simulink model "deltaM"  (Simulink 5.0)
settings: Solver=ode45  StartTime=0.0  StopTime=3  RelTol=1e-3
libraries: dspbuff3 x2, dspwin32 x2, dsparch4 x1
settings Model: LastModifiedBy=Daiming Qu

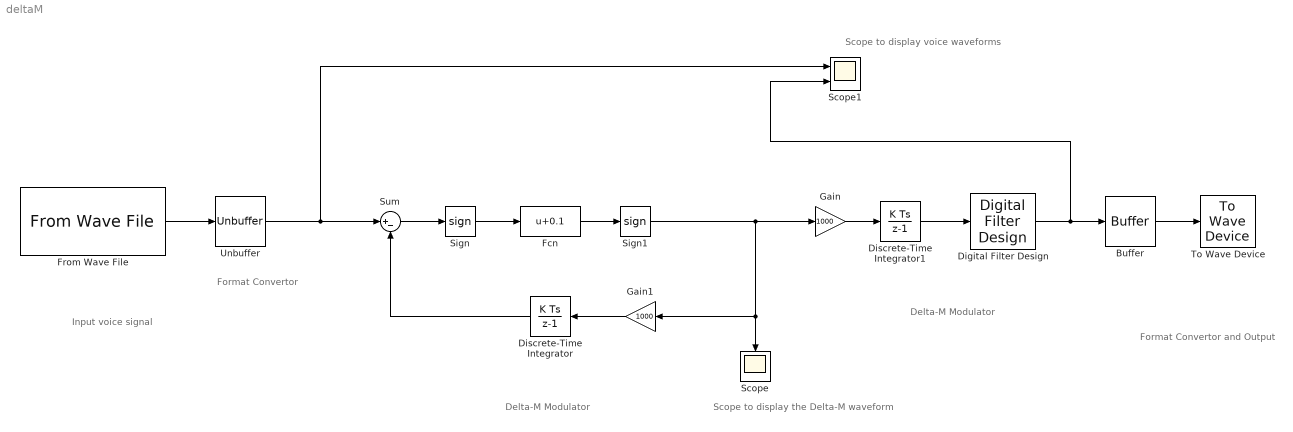
== system deltaM ==
  note: Format Convertor
  note: Scope to display voice waveforms
  note: Scope to display the
      | Delta-M waveform
  note: Format Convertor and Output
  note: Input voice signal
  note: Delta-M Modulator
  note: Delta-M Modulator
  Buffer : dspbuff3/Buffer  N=256  V=0  ic=0
  Digital Filter Design : dsparch4/Digital Filter Design
  Discrete-Time Integrator : DiscreteIntegrator  Orientation=left  SampleTime=-1
  Discrete-Time Integrator1 : DiscreteIntegrator  SampleTime=-1
  Fcn : Fcn  Expr=u+0.1
  From Wave File : dspwin32/From Wave File  FileName=speech_dian.wav  SamplesPerFrame=256  MinBufSize=256  dType=Double
  Gain : Gain  Gain=1000  SaturateOnIntegerOverflow=on
      settings: AttributesFormatString=Gain= %<Gain>
  Gain1 : Gain  Orientation=left  Gain=1000  SaturateOnIntegerOverflow=on
      settings: AttributesFormatString=Gain= %<Gain>
  Scope : Scope
      settings: Orientation=down  TimeRange=0.0004096000000011202  YMin=310.197  YMax=311.835
  Scope1 : Scope  NumInputPorts=2
      settings: TimeRange=10  YMin=-0.75~-0.75  YMax=1~0.75  SampleInput=on
  Sign : Signum
  Sign1 : Signum
  Sum : Sum  Inputs=|+-  SaturateOnIntegerOverflow=on
  To Wave Device : dspwin32/To Wave Device  bufDuration=2  initDelay=0.1  useDefaultDevice=on  userDeviceID=SoundMAX Digital Audio  enable24Bit=off
  Unbuffer : dspbuff3/Unbuffer  ic=0
  wires:
  Sum/1 -> Sign/1
  Discrete-Time Integrator/1 -> Sum/2
  Buffer/1 -> To Wave Device/1
  Discrete-Time Integrator1/1 -> Digital Filter Design/1
  Digital Filter Design/1 -> Buffer/1, Scope1/2
  Unbuffer/1 -> Sum/1, Scope1/1
  From Wave File/1 -> Unbuffer/1
  Sign/1 -> Fcn/1
  Fcn/1 -> Sign1/1
  Sign1/1 -> Scope/1, Gain1/1, Gain/1
  Gain/1 -> Discrete-Time Integrator1/1
  Gain1/1 -> Discrete-Time Integrator/1
